simulink model "RBL1"  (R2019a)
settings: Solver=VariableStepAuto  StartTime=0.0  StopTime=100  RelTol=1e-3
libraries: simulink x4
settings Model: Creator=Hariharan  LastModifiedBy=Hariharan
settings SolverCC: ZeroCrossAlgorithm=Adaptive
settings DebuggingCC: IgnoredZcDiagnostic=none

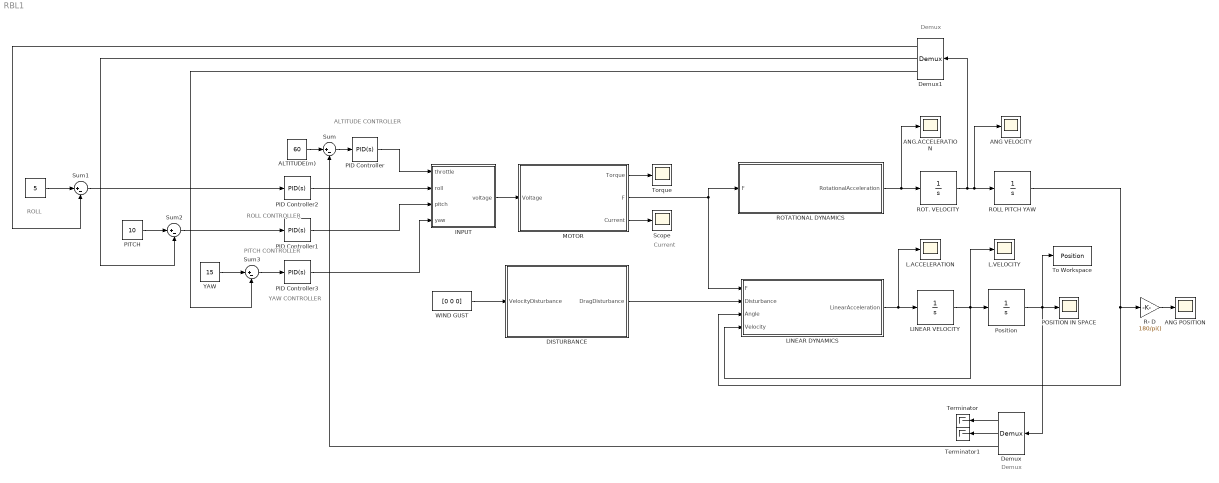
== system RBL1 ==
  note: Demux
  note: ALTITUDE CONTROLLER
  note: YAW CONTROLLER
  note: PITCH CONTROLLER
  note: ROLL CONTROLLER
  note: ROLL
  note: Current
  note: Demux
  "\tANG.ACCELERATION" : Scope
  "\tPOSITION IN SPACE" : Scope
  " " : Constant  Value=5
  ALTITUDE(m) : Constant  Value=60
  ANG POSITION : Scope
  ANG VELOCITY : Scope
  DISTURBANCE : MATLAB Function  TreatAsAtomicUnit=on
  Demux : Demux  Outputs=3
  Demux1 : Demux  Outputs=3
  INPUT : MATLAB Function  TreatAsAtomicUnit=on
  L.ACCELERATION : Scope
  L.VELOCITY : Scope
  LINEAR DYNAMICS : MATLAB Function  TreatAsAtomicUnit=on
  LINEAR VELOCITY : Integrator
  MOTOR : MATLAB Function  TreatAsAtomicUnit=on
  PID Controller : simulink/Continuous/PID Controller  Controller=PID  Form=Parallel  TimeDomain=Continuous-time  SampleTime=-1  IntegratorMethod=Forward Euler  FilterMethod=Forward Euler  ControllerParametersSource=internal  P=0.31  I=0.035  D=0.940835981825557  UseFilter=on  N=1142.8279760416  TunerSelectOption=Transfer Function Based (PID Tuner App)  InitialConditionSource=internal  InitialConditionForIntegrator=0  InitialConditionForFilter=0  DifferentiatorICPrevScaledInput=0  ExternalReset=none  TrackingMode=off  Kt=1  LimitOutput=on  UpperSaturationLimit=100  LowerSaturationLimit=0  LinearizeAsGain=on  AntiWindupMode=clamping  Kb=1  POutMin=[]  POutMax=[]  IOutMin=[]  IOutMax=[]  DOutMin=[]  DOutMax=[]  NOutMin=[]  NOutMax=[]  SumOutMin=[]  SumOutMax=[]  SaturationOutMin=[]  SaturationOutMax=[]  PParamMin=[]  PParamMax=[]  IParamMin=[]  IParamMax=[]  DParamMin=[]  DParamMax=[]  NParamMin=[]  NParamMax=[]  KbParamMin=[]  KbParamMax=[]  KtParamMin=[]  KtParamMax=[]  KbOutMin=[]  KbOutMax=[]  KtOutMin=[]  KtOutMax=[]  IntegratorOutMin=[]  IntegratorOutMax=[]  FilterOutMin=[]  FilterOutMax=[]  SumI1OutMin=[]  SumI1OutMax=[]  SumI2OutMin=[]  SumI2OutMax=[]  SumI3OutMin=[]  SumI3OutMax=[]  SumI4OutMin=[]  SumI4OutMax=[]  SumDOutMin=[]  SumDOutMax=[]  DifferentiatorOutMin=[]  DifferentiatorOutMax=[]  FilterDiffOutCoefMin=[]  FilterDiffOutCoefMax=[]  ReciprocalOutMin=[]  ReciprocalOutMax=[]  SumDenOutMin=[]  SumDenOutMax=[]  SumNumOutMin=[]  SumNumOutMax=[]  DivideOutMin=[]  DivideOutMax=[]  IntegratorContinuousStateAttributes=''  IntegratorStateMustResolveToSignalObject=off  IntegratorRTWStateStorageClass=Auto  FilterContinuousStateAttributes=''  FilterStateMustResolveToSignalObject=off  FilterRTWStateStorageClass=Auto  ParallelPVariant=InternalParameters  IdealPVariant=Disabled  IVariant=InternalParameters  DVariant=InternalParameters  IntegratorVariant=Continuous  SatVariant=Enabled  AWVariant=ContClampingParallel  PCopyVariant=Disabled  TRVariant=Disabled  FdbkBlocksVariant=Forward  IdealPFdbkVariant=Disabled  SatFdbkVariant=Disabled  DerivativeFilterVariant=ContFilter  NVariant=InternalParameters  NCopyVariant=Disabled  FilterICVariant=InternalICsFilter  IntegratorICVariant=InternalICs  ExternalResetVariant=Disabled  TRSumVariant=Passthrough  SumFdbkVariant=Disabled  SumVariant=Sum_PID
  PID Controller1 : simulink/Continuous/PID Controller  Controller=PID  Form=Parallel  TimeDomain=Continuous-time  SampleTime=-1  IntegratorMethod=Forward Euler  FilterMethod=Forward Euler  ControllerParametersSource=internal  P=0.2  I=0.00577686051048525  D=0.00714195620020144  UseFilter=on  N=5.51969158732913  TunerSelectOption=Transfer Function Based (PID Tuner App)  InitialConditionSource=internal  InitialConditionForIntegrator=0  InitialConditionForFilter=0  DifferentiatorICPrevScaledInput=0  ExternalReset=none  TrackingMode=off  Kt=1  LimitOutput=on  UpperSaturationLimit=100  LowerSaturationLimit=0  LinearizeAsGain=on  AntiWindupMode=clamping  Kb=1  POutMin=[]  POutMax=[]  IOutMin=[]  IOutMax=[]  DOutMin=[]  DOutMax=[]  NOutMin=[]  NOutMax=[]  SumOutMin=[]  SumOutMax=[]  SaturationOutMin=[]  SaturationOutMax=[]  PParamMin=[]  PParamMax=[]  IParamMin=[]  IParamMax=[]  DParamMin=[]  DParamMax=[]  NParamMin=[]  NParamMax=[]  KbParamMin=[]  KbParamMax=[]  KtParamMin=[]  KtParamMax=[]  KbOutMin=[]  KbOutMax=[]  KtOutMin=[]  KtOutMax=[]  IntegratorOutMin=[]  IntegratorOutMax=[]  FilterOutMin=[]  FilterOutMax=[]  SumI1OutMin=[]  SumI1OutMax=[]  SumI2OutMin=[]  SumI2OutMax=[]  SumI3OutMin=[]  SumI3OutMax=[]  SumI4OutMin=[]  SumI4OutMax=[]  SumDOutMin=[]  SumDOutMax=[]  DifferentiatorOutMin=[]  DifferentiatorOutMax=[]  FilterDiffOutCoefMin=[]  FilterDiffOutCoefMax=[]  ReciprocalOutMin=[]  ReciprocalOutMax=[]  SumDenOutMin=[]  SumDenOutMax=[]  SumNumOutMin=[]  SumNumOutMax=[]  DivideOutMin=[]  DivideOutMax=[]  IntegratorContinuousStateAttributes=''  IntegratorStateMustResolveToSignalObject=off  IntegratorRTWStateStorageClass=Auto  FilterContinuousStateAttributes=''  FilterStateMustResolveToSignalObject=off  FilterRTWStateStorageClass=Auto  ParallelPVariant=InternalParameters  IdealPVariant=Disabled  IVariant=InternalParameters  DVariant=InternalParameters  IntegratorVariant=Continuous  SatVariant=Enabled  AWVariant=ContClampingParallel  PCopyVariant=Disabled  TRVariant=Disabled  FdbkBlocksVariant=Forward  IdealPFdbkVariant=Disabled  SatFdbkVariant=Disabled  DerivativeFilterVariant=ContFilter  NVariant=InternalParameters  NCopyVariant=Disabled  FilterICVariant=InternalICsFilter  IntegratorICVariant=InternalICs  ExternalResetVariant=Disabled  TRSumVariant=Passthrough  SumFdbkVariant=Disabled  SumVariant=Sum_PID
  PID Controller2 : simulink/Continuous/PID Controller  Controller=PID  Form=Parallel  TimeDomain=Continuous-time  SampleTime=-1  IntegratorMethod=Forward Euler  FilterMethod=Forward Euler  ControllerParametersSource=internal  P=1  I=0.00577686051048525  D=0.00714195620020144  UseFilter=on  N=9.26685291207539  TunerSelectOption=Transfer Function Based (PID Tuner App)  InitialConditionSource=internal  InitialConditionForIntegrator=0  InitialConditionForFilter=0  DifferentiatorICPrevScaledInput=0  ExternalReset=none  TrackingMode=off  Kt=1  LimitOutput=on  UpperSaturationLimit=100  LowerSaturationLimit=0  LinearizeAsGain=on  AntiWindupMode=clamping  Kb=1  POutMin=[]  POutMax=[]  IOutMin=[]  IOutMax=[]  DOutMin=[]  DOutMax=[]  NOutMin=[]  NOutMax=[]  SumOutMin=[]  SumOutMax=[]  SaturationOutMin=[]  SaturationOutMax=[]  PParamMin=[]  PParamMax=[]  IParamMin=[]  IParamMax=[]  DParamMin=[]  DParamMax=[]  NParamMin=[]  NParamMax=[]  KbParamMin=[]  KbParamMax=[]  KtParamMin=[]  KtParamMax=[]  KbOutMin=[]  KbOutMax=[]  KtOutMin=[]  KtOutMax=[]  IntegratorOutMin=[]  IntegratorOutMax=[]  FilterOutMin=[]  FilterOutMax=[]  SumI1OutMin=[]  SumI1OutMax=[]  SumI2OutMin=[]  SumI2OutMax=[]  SumI3OutMin=[]  SumI3OutMax=[]  SumI4OutMin=[]  SumI4OutMax=[]  SumDOutMin=[]  SumDOutMax=[]  DifferentiatorOutMin=[]  DifferentiatorOutMax=[]  FilterDiffOutCoefMin=[]  FilterDiffOutCoefMax=[]  ReciprocalOutMin=[]  ReciprocalOutMax=[]  SumDenOutMin=[]  SumDenOutMax=[]  SumNumOutMin=[]  SumNumOutMax=[]  DivideOutMin=[]  DivideOutMax=[]  IntegratorContinuousStateAttributes=''  IntegratorStateMustResolveToSignalObject=off  IntegratorRTWStateStorageClass=Auto  FilterContinuousStateAttributes=''  FilterStateMustResolveToSignalObject=off  FilterRTWStateStorageClass=Auto  ParallelPVariant=InternalParameters  IdealPVariant=Disabled  IVariant=InternalParameters  DVariant=InternalParameters  IntegratorVariant=Continuous  SatVariant=Enabled  AWVariant=ContClampingParallel  PCopyVariant=Disabled  TRVariant=Disabled  FdbkBlocksVariant=Forward  IdealPFdbkVariant=Disabled  SatFdbkVariant=Disabled  DerivativeFilterVariant=ContFilter  NVariant=InternalParameters  NCopyVariant=Disabled  FilterICVariant=InternalICsFilter  IntegratorICVariant=InternalICs  ExternalResetVariant=Disabled  TRSumVariant=Passthrough  SumFdbkVariant=Disabled  SumVariant=Sum_PID
  PID Controller3 : simulink/Continuous/PID Controller  Controller=PID  Form=Parallel  TimeDomain=Continuous-time  SampleTime=-1  IntegratorMethod=Forward Euler  FilterMethod=Forward Euler  ControllerParametersSource=internal  P=1  I=0.00577686051048525  D=0.00714195620020144  UseFilter=on  N=5.51969158732913  TunerSelectOption=Transfer Function Based (PID Tuner App)  InitialConditionSource=internal  InitialConditionForIntegrator=0  InitialConditionForFilter=0  DifferentiatorICPrevScaledInput=0  ExternalReset=none  TrackingMode=off  Kt=1  LimitOutput=on  UpperSaturationLimit=100  LowerSaturationLimit=0  LinearizeAsGain=on  AntiWindupMode=clamping  Kb=1  POutMin=[]  POutMax=[]  IOutMin=[]  IOutMax=[]  DOutMin=[]  DOutMax=[]  NOutMin=[]  NOutMax=[]  SumOutMin=[]  SumOutMax=[]  SaturationOutMin=[]  SaturationOutMax=[]  PParamMin=[]  PParamMax=[]  IParamMin=[]  IParamMax=[]  DParamMin=[]  DParamMax=[]  NParamMin=[]  NParamMax=[]  KbParamMin=[]  KbParamMax=[]  KtParamMin=[]  KtParamMax=[]  KbOutMin=[]  KbOutMax=[]  KtOutMin=[]  KtOutMax=[]  IntegratorOutMin=[]  IntegratorOutMax=[]  FilterOutMin=[]  FilterOutMax=[]  SumI1OutMin=[]  SumI1OutMax=[]  SumI2OutMin=[]  SumI2OutMax=[]  SumI3OutMin=[]  SumI3OutMax=[]  SumI4OutMin=[]  SumI4OutMax=[]  SumDOutMin=[]  SumDOutMax=[]  DifferentiatorOutMin=[]  DifferentiatorOutMax=[]  FilterDiffOutCoefMin=[]  FilterDiffOutCoefMax=[]  ReciprocalOutMin=[]  ReciprocalOutMax=[]  SumDenOutMin=[]  SumDenOutMax=[]  SumNumOutMin=[]  SumNumOutMax=[]  DivideOutMin=[]  DivideOutMax=[]  IntegratorContinuousStateAttributes=''  IntegratorStateMustResolveToSignalObject=off  IntegratorRTWStateStorageClass=Auto  FilterContinuousStateAttributes=''  FilterStateMustResolveToSignalObject=off  FilterRTWStateStorageClass=Auto  ParallelPVariant=InternalParameters  IdealPVariant=Disabled  IVariant=InternalParameters  DVariant=InternalParameters  IntegratorVariant=Continuous  SatVariant=Enabled  AWVariant=ContClampingParallel  PCopyVariant=Disabled  TRVariant=Disabled  FdbkBlocksVariant=Forward  IdealPFdbkVariant=Disabled  SatFdbkVariant=Disabled  DerivativeFilterVariant=ContFilter  NVariant=InternalParameters  NCopyVariant=Disabled  FilterICVariant=InternalICsFilter  IntegratorICVariant=InternalICs  ExternalResetVariant=Disabled  TRSumVariant=Passthrough  SumFdbkVariant=Disabled  SumVariant=Sum_PID
  "PITCH " : Constant  Value=10
  Position : Integrator
  R- D : Gain  Gain=180/pi()
  ROLL PITCH YAW : Integrator
  ROT. VELOCITY : Integrator
  ROTATIONAL DYNAMICS : MATLAB Function  TreatAsAtomicUnit=on
  Scope : Scope
  Sum{,1..3} (4 alike) : Sum  Inputs=|+-
  Terminator : Terminator
  Terminator1 : Terminator
  To Workspace : ToWorkspace  VariableName=Position  SampleTime=-1
      settings: Save2DSignal=2-D array (concatenate along first dimension)
  Torque : Scope
  WIND GUST : Constant  Value=[0 0 0]
  YAW : Constant  Value=15
  wires:
  MOTOR/2(F) -> ROTATIONAL DYNAMICS/1(F), LINEAR DYNAMICS/1(F)
  ROTATIONAL DYNAMICS/1(RotationalAcceleration) -> "\tANG.ACCELERATION"/1, ROT. VELOCITY/1
  LINEAR DYNAMICS/1(LinearAcceleration) -> L.ACCELERATION/1, LINEAR VELOCITY/1
  LINEAR VELOCITY/1 -> L.VELOCITY/1, LINEAR DYNAMICS/4(Velocity), Position/1
  DISTURBANCE/1(DragDisturbance) -> LINEAR DYNAMICS/2(Disturbance)
  WIND GUST/1 -> DISTURBANCE/1(VelocityDisturbance)
  INPUT/1(voltage) -> MOTOR/1(Voltage)
  PID Controller3/1 -> INPUT/4(yaw)
  R- D/1 -> ANG POSITION/1
  MOTOR/3(Current) -> Scope/1
  Position/1 -> Demux/1, To Workspace/1, "\tPOSITION IN SPACE"/1
  PID Controller/1 -> INPUT/1(throttle)
  ALTITUDE(m)/1 -> Sum/1
  Sum/1 -> PID Controller/1
  Demux/3 -> Sum/2
  Demux/1 -> Terminator/1
  Demux/2 -> Terminator1/1
  ROT. VELOCITY/1 -> Demux1/1, ANG VELOCITY/1, ROLL PITCH YAW/1
  ROLL PITCH YAW/1 -> R- D/1, LINEAR DYNAMICS/3(Angle)
  MOTOR/1(Torque) -> Torque/1
  PID Controller2/1 -> INPUT/2(roll)
  "PITCH "/1 -> Sum2/1
  Sum2/1 -> PID Controller1/1
  PID Controller1/1 -> INPUT/3(pitch)
  Demux1/2 -> Sum2/2
  Sum1/1 -> PID Controller2/1
  " "/1 -> Sum1/1
  Demux1/1 -> Sum1/2
  Sum3/1 -> PID Controller3/1
  YAW/1 -> Sum3/1
  Demux1/3 -> Sum3/2

== matlab function RBL1/ROTATIONAL DYNAMICS ==
  data: RotationalAcceleration output; F input
% function RotationalAcceleration = fcn(Torque,F)
% Moment=[0 0 0 0];
% Inertia=[0.003 0.003 0.007];
% RotationalAcceleration=[0 0 0];
% Moment(1)=(F(3)+F(4))*0.237/2-(F(1)+F(2))*0.237/2;
% Moment(2)=(F(3)+F(2))*0.237/2-(F(1)+F(4))*0.237/2;
% Moment(3)=Torque(4)-Torque(1)+Torque(2)-Torque(3);
% Moment(4) = F(1)+F(2)+F(3)+F(4);
% for i=1:3
%     RotationalAcceleration(i)=Moment(i)/Inertia(i);
% end
function RotationalAcceleration = fcn(F)
Moment=[0 0 0 0];
Inertia=[0.003 0.003 0.007];
RotationalAcceleration=[0 0 0];
Moment(1)=(F(4)-F(2))*0.237/2;
Moment(2)=(F(3)-F(1))*0.237/2;
Moment(3)=F(4)-F(1)+F(2)-F(3);
Moment(4) = F(1)+F(2)+F(3)+F(4);
for i=1:3
    RotationalAcceleration(i)=Moment(i)/Inertia(i);
end

% function RotationalAcceleration = fcn(Torque,F)
% Moment=[0 0 0 0];
% Inertia=[0.003 0.003 0.007];
% RotationalAcceleration=[0 0 0];
% Moment(1)=(Torque(4)-Torque(2))*0.237/2;
% Moment(2)=(Torque(3)-Torque(1))*0.237/2;
% Moment(3)=Torque(4)-Torque(1)+Torque(2)-Torque(3);
% Moment(4) = F(1)+F(2)+F(3)+F(4);
% for i=1:3
%     RotationalAcceleration(i)=Moment(i)/Inertia(i);
% end

== matlab function RBL1/MOTOR ==
  data: Voltage input; Torque output; F output; Current output
function [Torque, F, Current] = fcn(Voltage)
RPM=[0 0 0 0];
Torque=[0 0 0 0 0];
Current=[0 0 0 0];
F=[0 0 0 0];
for i=1:4
    RPM(i)=-62*Voltage(i)^2+2750*Voltage(i);
    Ct=4*10^-15*RPM(i)^3+3*10^-10*RPM(i)^2-4*10^-6*RPM(i)+0.1983;
    F(i)=Ct*1.225*(RPM(i)/60)^2*0.2^4;
    Torque(i)=-4*10^-14*RPM(i)^3+4*10^-9*RPM(i)^2-7*10^-5*RPM(i)+0.3534;
    Current(i)=1400*Torque(i);
end

== matlab function RBL1/LINEAR DYNAMICS ==
  data: F input; Disturbance input; Angle input; Velocity input; LinearAcceleration output
function LinearAcceleration  = fcn(F,Disturbance, Angle, Velocity)
m = 0.743;
g = 9.81;
area= [0.0197 0.0197 0.0512];
adensity = 1.225;
cd = 1;
LinearAcceleration = [0 0 0];
Force = [0 0 0];
FProp = [0 0 0];
FProp(1) = ((sin(Angle(1))* sin(Angle(3))) + (cos(Angle(1)) * sin(Angle(2)) * cos(Angle(3))))*(F(1)+F(2)+F(3)+F(4));

FProp(2) = ((cos(Angle(1))* sin(Angle(2)) * sin(Angle(3)))  -  (sin(Angle(1)) * cos(Angle(3))))*(F(1)+F(2)+F(3)+F(4));
FProp(3) = (1)*(F(1)+F(2)+F(3)+F(4));

if(Velocity(1) < 0)
    Force(1) = FProp(1) - Disturbance(1) + 0.5*adensity*Velocity(1)^2*area(1)*cd;
else
    Force(1) = FProp(1) - Disturbance(1) - 0.5*adensity*Velocity(1)^2*area(1)*cd;
end
if(Velocity(2) < 0)
    Force(2) = FProp(2) - Disturbance(2) + 0.5*adensity*Velocity(2)^2*area(2)*cd;
else
    Force(2) = FProp(2) - Disturbance(2) - 0.5*adensity*Velocity(2)^2*area(2)*cd;
end
if(Velocity(3) < 0)
    Force(3) =  FProp(3) - Disturbance(3) + 0.5*adensity*Velocity(3)^2*area(3)*cd - (m * g) ;
else
    Force(3) = FProp(3) - Disturbance(3) - 0.5*adensity*Velocity(3)^2*area(3)*cd - (m * g) ;
end
for i=1:3
    LinearAcceleration(i) = Force(i)/m;
end

== matlab function RBL1/DISTURBANCE ==
  data: VelocityDisturbance input; DragDisturbance output
function DragDisturbance  = fcn(VelocityDisturbance)

area= [0.0197 0.0197 0.0512];
DragDisturbance = [0 0 0];
adensity = 1.225;
cd =1;
for i=1:3
    if VelocityDisturbance(i)<0
        DragDisturbance(i)=0.5*adensity*VelocityDisturbance(i)^2*area(i)*cd;
    else
        DragDisturbance(i)=-0.5*adensity*VelocityDisturbance(i)^2*area(i)*cd;
    end
end

== matlab function RBL1/INPUT ==
  data: throttle input; roll input; pitch input; voltage output; yaw input
function voltage = fcn(throttle,roll,pitch,yaw)
correct = 0;
if(roll/2+pitch/2+yaw/2 > (100 - throttle))
    correct = ((roll/2+pitch/2+yaw/2)-(100-throttle));
end
if(roll/2+pitch/2+yaw/2 > throttle)
    if correct < (roll/2+pitch/2+yaw/2 - throttle)
        correct = (roll/2+pitch/2+yaw/2 - throttle);
    end
end
roll = (roll - correct / 3) *2;
pitch = (pitch - correct / 3) *2;
yaw = (yaw - correct / 3) *2;
voltage = [(((throttle - roll/2 - pitch/2 - yaw/2) * 11.4) / 100)
    (((throttle - roll/2 + pitch/2 + yaw/2) * 11.4) / 100)
    (((throttle + roll/2 + pitch/2 - yaw/2) * 11.4) / 100)
    (((throttle + roll/2 - pitch/2 + yaw/2) * 11.4) / 100)];
